simulink model "test_simple_update_gen"  (Simulink 7.7)
settings: Solver=FixedStepDiscrete  StartTime=0.0  StopTime=10000.0  FixedStep=1  RelTol=1e-3
libraries: SimpleModeling x2
settings Model: Creator=medcps  LastModifiedBy=iris
settings DataIOCC: SaveFormat=Structure
settings OptimizationCC: BlockReduction=off  ConditionallyExecuteInputs=off
settings DebuggingCC: FcnCallInpInsideContextMsg=Enable All

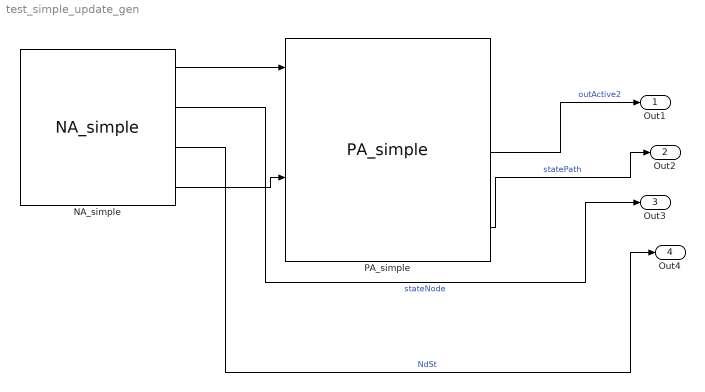
== system test_simple_update_gen ==
  NA_simple : SimpleModeling/NA_simple  SystemSampleTime=-1  TERP_defs=0  TRRP_def=100  Trest_def=800  TERP_start=320  TRRP_start=100  Trest_start=800  Terp_min=150  Terp_max=300
  PA_simple : SimpleModeling/PA_simple  SystemSampleTime=-1  forw_timer_defs=22  bck_timer_defs=22  min_path_par=22  bck_param=2  forw_param=2
  Out1 : Outport
  Out2 : Outport  Port=2
  Out3 : Outport  Port=3
  Out4 : Outport  Port=4
  wires:
  NA_simple/1 -> PA_simple/1
  NA_simple/3 -> Out4/1  "NdSt"
  PA_simple/2 -> Out1/1  "outActive2"
  PA_simple/3 -> Out2/1  "statePath"
  NA_simple/2 -> Out3/1  "stateNode"
  NA_simple/4 -> PA_simple/3
